simulink model "Partie_03"  (R2020a)
settings: Solver=FixedStepAuto  StartTime=0.0  StopTime=1e-3  FixedStep=Ts  RelTol=1e-3
values from neighbouring files (symbols this model uses):
  A = 15*1e-6    (= 1.5e-05)    [TP_Linear_I.m]
  Kamp = 10    [TP_Linear_I.m]
  ke = 0.3    [TP_Linear_I.m]
  W = 2*pi*F    (= 6283.18530718)    [TP_Linear_I.m]
libraries: cstblocks x2
settings Model: Creator=mehdi  LastModifiedBy=mehdi

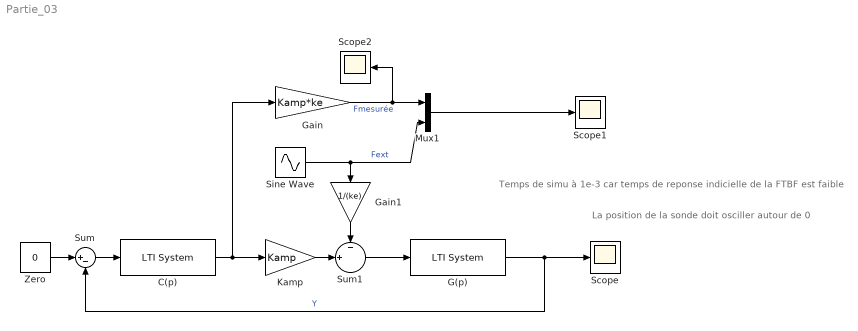
== system Partie_03 ==
  note: Temps de simu à 1e-3 car temps de reponse indicielle de la FTBF est faible
  note: La position de la sonde doit osciller autour de 0
  C(p) : cstblocks/LTI System  sys=C  IC=[]
  G(p) : cstblocks/LTI System  sys=G  IC=[]
  Gain : Gain  Gain=Kamp*ke
  Gain1 : Gain  Gain=1/(ke)
  Kamp : Gain  Gain=Kamp
  Mux1 : Mux  Inputs=2
  Scope : Scope
  Scope1 : Scope
  Scope2 : Scope
  Sine Wave : Sin  Amplitude=A  Frequency=W  SampleTime=0
  Sum : Sum  Inputs=|+-
  Sum1 : Sum  Inputs=-|+||
  Zero : Constant  Value=0  OutDataTypeStr=Inherit: Inherit via back propagation
  wires:
  Sum/1 -> C(p)/1
  C(p)/1 -> Kamp/1, Gain/1
  Kamp/1 -> Sum1/2
  Sum1/1 -> G(p)/1
  Gain1/1 -> Sum1/1
  G(p)/1 -> Scope/1, Sum/2  "Y"
  Sine Wave/1 -> Gain1/1, Mux1/2  "Fext"
  Zero/1 -> Sum/1
  Mux1/1 -> Scope1/1
  Gain/1 -> Scope2/1, Mux1/1  "Fmesurée"
